simulink model "controlGPI_pos_6dof_conMI"  (R2023b)
settings: Solver=ode45  StartTime=0.0  StopTime=tsim  FixedStep=1e-4  MaxStep=tstep
undefined symbols (not defined in the file): contr_robot_params, ddq, dq, MI_Contr1, MI_Contr2, MI_Contr3, MI_Contr4, MI_Contr5, MI_Contr6, MI_motor1, MI_motor2, MI_motor3, MI_motor4, MI_motor5, MI_motor6, ndof, NN_Bspline_params, NN_RBF_params, nn_select, ns, Pc, q0, q_cero, q_eq, robot_params, sigbuilder_block, t_qeq_init, t_tr_init, t_trtr, tau_L, tau_L_mags, tr_muestra, tr_ref, Wc, Zc
libraries: mcbcontrolslib x12, spsRMSLib x12, simulink x2
(part 2 of 4)

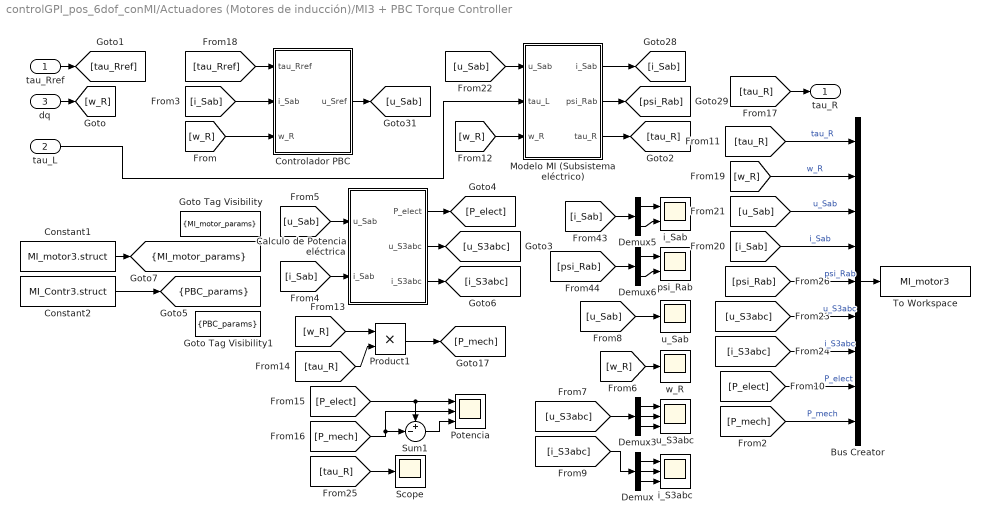
== system controlGPI_pos_6dof_conMI/Actuadores (Motores de inducción)/MI3 + PBC Torque Controller ==
  tau_Rref : Inport
  tau_L : Inport  Port=2
  dq : Inport  Port=3
  Bus Creator : BusCreator  Inputs=9
  Calculo de Potencia eléctrica : Subsystem
  Constant1 : Constant  Value=MI_motor3.struct  OutDataTypeStr=Bus: MI_bus
  Constant2 : Constant  Value=MI_Contr3.struct  OutDataTypeStr=Bus: Contr_bus
  Controlador PBC : Subsystem
  Demux : Demux  Outputs=3
  Demux3 : Demux  Outputs=3
  Demux5 : Demux  Outputs=2
  Demux6 : Demux  Outputs=2
  Goto Tag Visibility : GotoTagVisibility  GotoTag=MI_motor_params
  Goto Tag Visibility1 : GotoTagVisibility  GotoTag=PBC_params
  Modelo MI (Subsistema eléctrico) : Subsystem
  Potencia : Scope  NumInputPorts=3
  Product1 : Product
  Scope : Scope
  Sum1 : Sum  Inputs=+-|
  To Workspace : ToWorkspace  VariableName=MI_motor3  SaveFormat=Timeseries  SampleTime=-1
  i_S3abc : Scope  NumInputPorts=3
  i_Sab : Scope  NumInputPorts=2
  psi_Rab : Scope  NumInputPorts=2
  u_S3abc : Scope  NumInputPorts=3
  u_Sab : Scope
  w_R : Scope
  tau_R : Outport
  tag scope: MI_motor_params=scoped, PBC_params=scoped
  wires:
  Modelo MI (Subsistema eléctrico)/2(psi_Rab) -> [psi_Rab]
  [u_Sab] -> Modelo MI (Subsistema eléctrico)/1(u_Sab)
  [i_Sab] -> Controlador PBC/2(i_Sab)
  Controlador PBC/1(u_Sref) -> [u_Sab]
  [w_R] -> Controlador PBC/3(w_R)
  Calculo de Potencia eléctrica/2(u_S3abc) -> [u_S3abc]
  Calculo de Potencia eléctrica/1(P_elect) -> [P_elect]
  Demux5/1 -> i_Sab/1
  [w_R] -> w_R/1
  [u_Sab] -> Calculo de Potencia eléctrica/1(u_Sab)
  [psi_Rab] -> Demux6/1
  [u_Sab] -> u_Sab/1
  Demux6/1 -> psi_Rab/1
  Calculo de Potencia eléctrica/3(i_S3abc) -> [i_S3abc]
  Demux6/2 -> psi_Rab/2
  Demux5/2 -> i_Sab/2
  [i_Sab] -> Calculo de Potencia eléctrica/2(i_Sab)
  [i_Sab] -> Demux5/1
  Demux/2 -> i_S3abc/2
  Demux3/1 -> u_S3abc/1
  Demux3/3 -> u_S3abc/3
  [i_S3abc] -> Demux/1
  Demux/1 -> i_S3abc/1
  Demux/3 -> i_S3abc/3
  [u_S3abc] -> Demux3/1
  Demux3/2 -> u_S3abc/2
  Modelo MI (Subsistema eléctrico)/1(i_Sab) -> [i_Sab]
  Modelo MI (Subsistema eléctrico)/3(tau_R) -> [tau_R]
  Product1/1 -> [P_mech]
  [w_R] -> Product1/1
  [tau_R] -> Product1/2
  [tau_R] -> Bus Creator/1  "tau_R"
  Sum1/1 -> Potencia/3
  [P_elect] -> Potencia/1, Sum1/1
  [P_mech] -> Potencia/2, Sum1/2
  [tau_R] -> tau_R/1
  dq/1 -> [w_R]
  [tau_Rref] -> Controlador PBC/1(tau_Rref)
  [w_R] -> Modelo MI (Subsistema eléctrico)/3(w_R)
  Bus Creator/1 -> To Workspace/1
  Constant1/1 -> [MI_motor_params]
  [tau_R] -> Scope/1
  Constant2/1 -> [PBC_params]
  [w_R] -> Bus Creator/2  "w_R"
  [u_Sab] -> Bus Creator/3  "u_Sab"
  [i_Sab] -> Bus Creator/4  "i_Sab"
  [u_S3abc] -> Bus Creator/6  "u_S3abc"
  [i_S3abc] -> Bus Creator/7  "i_S3abc"
  [P_elect] -> Bus Creator/8  "P_elect"
  [P_mech] -> Bus Creator/9  "P_mech"
  tau_Rref/1 -> [tau_Rref]
  [psi_Rab] -> Bus Creator/5  "psi_Rab"
  tau_L/1 -> Modelo MI (Subsistema eléctrico)/2(tau_L)

== system controlGPI_pos_6dof_conMI/Actuadores (Motores de inducción)/MI4 + PBC Torque Controller ==
  tau_Rref : Inport
  tau_L : Inport  Port=2
  dq : Inport  Port=3
  Bus Creator : BusCreator  Inputs=9
  Calculo de Potencia eléctrica : Subsystem
  Constant1 : Constant  Value=MI_motor4.struct  OutDataTypeStr=Bus: MI_bus
  Constant2 : Constant  Value=MI_Contr4.struct  OutDataTypeStr=Bus: Contr_bus
  Controlador PBC : Subsystem
  Demux : Demux  Outputs=3
  Demux3 : Demux  Outputs=3
  Demux5 : Demux  Outputs=2
  Demux6 : Demux  Outputs=2
  Goto Tag Visibility : GotoTagVisibility  GotoTag=MI_motor_params
  Goto Tag Visibility1 : GotoTagVisibility  GotoTag=PBC_params
  Modelo MI (Subsistema eléctrico) : Subsystem
  Potencia : Scope  NumInputPorts=3
  Product1 : Product
  Scope : Scope
  Sum1 : Sum  Inputs=+-|
  To Workspace : ToWorkspace  VariableName=MI_motor4  SaveFormat=Timeseries  SampleTime=-1
  i_S3abc : Scope  NumInputPorts=3
  i_Sab : Scope  NumInputPorts=2
  psi_Rab : Scope  NumInputPorts=2
  u_S3abc : Scope  NumInputPorts=3
  u_Sab : Scope
  w_R : Scope
  tau_R : Outport
  tag scope: MI_motor_params=scoped, PBC_params=scoped
  wires:
  Modelo MI (Subsistema eléctrico)/2(psi_Rab) -> [psi_Rab]
  [u_Sab] -> Modelo MI (Subsistema eléctrico)/1(u_Sab)
  [i_Sab] -> Controlador PBC/2(i_Sab)
  Controlador PBC/1(u_Sref) -> [u_Sab]
  [w_R] -> Controlador PBC/3(w_R)
  Calculo de Potencia eléctrica/2(u_S3abc) -> [u_S3abc]
  Calculo de Potencia eléctrica/1(P_elect) -> [P_elect]
  Demux5/1 -> i_Sab/1
  [w_R] -> w_R/1
  [u_Sab] -> Calculo de Potencia eléctrica/1(u_Sab)
  [psi_Rab] -> Demux6/1
  [u_Sab] -> u_Sab/1
  Demux6/1 -> psi_Rab/1
  Calculo de Potencia eléctrica/3(i_S3abc) -> [i_S3abc]
  Demux6/2 -> psi_Rab/2
  Demux5/2 -> i_Sab/2
  [i_Sab] -> Calculo de Potencia eléctrica/2(i_Sab)
  [i_Sab] -> Demux5/1
  Demux/2 -> i_S3abc/2
  Demux3/1 -> u_S3abc/1
  Demux3/3 -> u_S3abc/3
  [i_S3abc] -> Demux/1
  Demux/1 -> i_S3abc/1
  Demux/3 -> i_S3abc/3
  [u_S3abc] -> Demux3/1
  Demux3/2 -> u_S3abc/2
  Modelo MI (Subsistema eléctrico)/1(i_Sab) -> [i_Sab]
  Modelo MI (Subsistema eléctrico)/3(tau_R) -> [tau_R]
  Product1/1 -> [P_mech]
  [w_R] -> Product1/1
  [tau_R] -> Product1/2
  [tau_R] -> Bus Creator/1  "tau_R"
  Sum1/1 -> Potencia/3
  [P_elect] -> Potencia/1, Sum1/1
  [P_mech] -> Potencia/2, Sum1/2
  [tau_R] -> tau_R/1
  dq/1 -> [w_R]
  [tau_Rref] -> Controlador PBC/1(tau_Rref)
  [w_R] -> Modelo MI (Subsistema eléctrico)/3(w_R)
  Bus Creator/1 -> To Workspace/1
  Constant1/1 -> [MI_motor_params]
  [tau_R] -> Scope/1
  Constant2/1 -> [PBC_params]
  [w_R] -> Bus Creator/2  "w_R"
  [u_Sab] -> Bus Creator/3  "u_Sab"
  [i_Sab] -> Bus Creator/4  "i_Sab"
  [u_S3abc] -> Bus Creator/6  "u_S3abc"
  [i_S3abc] -> Bus Creator/7  "i_S3abc"
  [P_elect] -> Bus Creator/8  "P_elect"
  [P_mech] -> Bus Creator/9  "P_mech"
  tau_Rref/1 -> [tau_Rref]
  [psi_Rab] -> Bus Creator/5  "psi_Rab"
  tau_L/1 -> Modelo MI (Subsistema eléctrico)/2(tau_L)

== system controlGPI_pos_6dof_conMI/Actuadores (Motores de inducción)/MI5 + PBC Torque Controller ==
  tau_Rref : Inport
  tau_L : Inport  Port=2
  dq : Inport  Port=3
  Bus Creator : BusCreator  Inputs=9
  Calculo de Potencia eléctrica : Subsystem
  Constant1 : Constant  Value=MI_motor5.struct  OutDataTypeStr=Bus: MI_bus
  Constant2 : Constant  Value=MI_Contr5.struct  OutDataTypeStr=Bus: Contr_bus
  Controlador PBC : Subsystem
  Demux : Demux  Outputs=3
  Demux3 : Demux  Outputs=3
  Demux5 : Demux  Outputs=2
  Demux6 : Demux  Outputs=2
  Goto Tag Visibility : GotoTagVisibility  GotoTag=MI_motor_params
  Goto Tag Visibility1 : GotoTagVisibility  GotoTag=PBC_params
  Modelo MI (Subsistema eléctrico) : Subsystem
  Potencia : Scope  NumInputPorts=3
  Product1 : Product
  Scope : Scope
  Sum1 : Sum  Inputs=+-|
  To Workspace : ToWorkspace  VariableName=MI_motor5  SaveFormat=Timeseries  SampleTime=-1
  i_S3abc : Scope  NumInputPorts=3
  i_Sab : Scope  NumInputPorts=2
  psi_Rab : Scope  NumInputPorts=2
  u_S3abc : Scope  NumInputPorts=3
  u_Sab : Scope
  w_R : Scope
  tau_R : Outport
  tag scope: MI_motor_params=scoped, PBC_params=scoped
  wires:
  Modelo MI (Subsistema eléctrico)/2(psi_Rab) -> [psi_Rab]
  [u_Sab] -> Modelo MI (Subsistema eléctrico)/1(u_Sab)
  [i_Sab] -> Controlador PBC/2(i_Sab)
  Controlador PBC/1(u_Sref) -> [u_Sab]
  [w_R] -> Controlador PBC/3(w_R)
  Calculo de Potencia eléctrica/2(u_S3abc) -> [u_S3abc]
  Calculo de Potencia eléctrica/1(P_elect) -> [P_elect]
  Demux5/1 -> i_Sab/1
  [w_R] -> w_R/1
  [u_Sab] -> Calculo de Potencia eléctrica/1(u_Sab)
  [psi_Rab] -> Demux6/1
  [u_Sab] -> u_Sab/1
  Demux6/1 -> psi_Rab/1
  Calculo de Potencia eléctrica/3(i_S3abc) -> [i_S3abc]
  Demux6/2 -> psi_Rab/2
  Demux5/2 -> i_Sab/2
  [i_Sab] -> Calculo de Potencia eléctrica/2(i_Sab)
  [i_Sab] -> Demux5/1
  Demux/2 -> i_S3abc/2
  Demux3/1 -> u_S3abc/1
  Demux3/3 -> u_S3abc/3
  [i_S3abc] -> Demux/1
  Demux/1 -> i_S3abc/1
  Demux/3 -> i_S3abc/3
  [u_S3abc] -> Demux3/1
  Demux3/2 -> u_S3abc/2
  Modelo MI (Subsistema eléctrico)/1(i_Sab) -> [i_Sab]
  Modelo MI (Subsistema eléctrico)/3(tau_R) -> [tau_R]
  Product1/1 -> [P_mech]
  [w_R] -> Product1/1
  [tau_R] -> Product1/2
  [tau_R] -> Bus Creator/1  "tau_R"
  Sum1/1 -> Potencia/3
  [P_elect] -> Potencia/1, Sum1/1
  [P_mech] -> Potencia/2, Sum1/2
  [tau_R] -> tau_R/1
  dq/1 -> [w_R]
  [tau_Rref] -> Controlador PBC/1(tau_Rref)
  [w_R] -> Modelo MI (Subsistema eléctrico)/3(w_R)
  Bus Creator/1 -> To Workspace/1
  Constant1/1 -> [MI_motor_params]
  [tau_R] -> Scope/1
  Constant2/1 -> [PBC_params]
  [w_R] -> Bus Creator/2  "w_R"
  [u_Sab] -> Bus Creator/3  "u_Sab"
  [i_Sab] -> Bus Creator/4  "i_Sab"
  [u_S3abc] -> Bus Creator/6  "u_S3abc"
  [i_S3abc] -> Bus Creator/7  "i_S3abc"
  [P_elect] -> Bus Creator/8  "P_elect"
  [P_mech] -> Bus Creator/9  "P_mech"
  tau_Rref/1 -> [tau_Rref]
  [psi_Rab] -> Bus Creator/5  "psi_Rab"
  tau_L/1 -> Modelo MI (Subsistema eléctrico)/2(tau_L)

== system controlGPI_pos_6dof_conMI/Actuadores (Motores de inducción)/MI6 + PBC Torque Controller ==
  tau_Rref : Inport
  tau_L : Inport  Port=2
  dq : Inport  Port=3
  Bus Creator : BusCreator  Inputs=9
  Calculo de Potencia eléctrica : Subsystem
  Constant1 : Constant  Value=MI_motor6.struct  OutDataTypeStr=Bus: MI_bus
  Constant2 : Constant  Value=MI_Contr6.struct  OutDataTypeStr=Bus: Contr_bus
  Controlador PBC : Subsystem
  Demux : Demux  Outputs=3
  Demux3 : Demux  Outputs=3
  Demux5 : Demux  Outputs=2
  Demux6 : Demux  Outputs=2
  Goto Tag Visibility : GotoTagVisibility  GotoTag=MI_motor_params
  Goto Tag Visibility1 : GotoTagVisibility  GotoTag=PBC_params
  Modelo MI (Subsistema eléctrico) : Subsystem
  Potencia : Scope  NumInputPorts=3
  Product1 : Product
  Scope : Scope
  Sum1 : Sum  Inputs=+-|
  To Workspace : ToWorkspace  VariableName=MI_motor6  SaveFormat=Timeseries  SampleTime=-1
  i_S3abc : Scope  NumInputPorts=3
  i_Sab : Scope  NumInputPorts=2
  psi_Rab : Scope  NumInputPorts=2
  u_S3abc : Scope  NumInputPorts=3
  u_Sab : Scope
  w_R : Scope
  tau_R : Outport
  tag scope: MI_motor_params=scoped, PBC_params=scoped
  wires:
  Modelo MI (Subsistema eléctrico)/2(psi_Rab) -> [psi_Rab]
  [u_Sab] -> Modelo MI (Subsistema eléctrico)/1(u_Sab)
  [i_Sab] -> Controlador PBC/2(i_Sab)
  Controlador PBC/1(u_Sref) -> [u_Sab]
  [w_R] -> Controlador PBC/3(w_R)
  Calculo de Potencia eléctrica/2(u_S3abc) -> [u_S3abc]
  Calculo de Potencia eléctrica/1(P_elect) -> [P_elect]
  Demux5/1 -> i_Sab/1
  [w_R] -> w_R/1
  [u_Sab] -> Calculo de Potencia eléctrica/1(u_Sab)
  [psi_Rab] -> Demux6/1
  [u_Sab] -> u_Sab/1
  Demux6/1 -> psi_Rab/1
  Calculo de Potencia eléctrica/3(i_S3abc) -> [i_S3abc]
  Demux6/2 -> psi_Rab/2
  Demux5/2 -> i_Sab/2
  [i_Sab] -> Calculo de Potencia eléctrica/2(i_Sab)
  [i_Sab] -> Demux5/1
  Demux/2 -> i_S3abc/2
  Demux3/1 -> u_S3abc/1
  Demux3/3 -> u_S3abc/3
  [i_S3abc] -> Demux/1
  Demux/1 -> i_S3abc/1
  Demux/3 -> i_S3abc/3
  [u_S3abc] -> Demux3/1
  Demux3/2 -> u_S3abc/2
  Modelo MI (Subsistema eléctrico)/1(i_Sab) -> [i_Sab]
  Modelo MI (Subsistema eléctrico)/3(tau_R) -> [tau_R]
  Product1/1 -> [P_mech]
  [w_R] -> Product1/1
  [tau_R] -> Product1/2
  [tau_R] -> Bus Creator/1  "tau_R"
  Sum1/1 -> Potencia/3
  [P_elect] -> Potencia/1, Sum1/1
  [P_mech] -> Potencia/2, Sum1/2
  [tau_R] -> tau_R/1
  dq/1 -> [w_R]
  [tau_Rref] -> Controlador PBC/1(tau_Rref)
  [w_R] -> Modelo MI (Subsistema eléctrico)/3(w_R)
  Bus Creator/1 -> To Workspace/1
  Constant1/1 -> [MI_motor_params]
  [tau_R] -> Scope/1
  Constant2/1 -> [PBC_params]
  [w_R] -> Bus Creator/2  "w_R"
  [u_Sab] -> Bus Creator/3  "u_Sab"
  [i_Sab] -> Bus Creator/4  "i_Sab"
  [u_S3abc] -> Bus Creator/6  "u_S3abc"
  [i_S3abc] -> Bus Creator/7  "i_S3abc"
  [P_elect] -> Bus Creator/8  "P_elect"
  [P_mech] -> Bus Creator/9  "P_mech"
  tau_Rref/1 -> [tau_Rref]
  [psi_Rab] -> Bus Creator/5  "psi_Rab"
  tau_L/1 -> Modelo MI (Subsistema eléctrico)/2(tau_L)

== system controlGPI_pos_6dof_conMI/ControladorGPI + NN/2 to 3 (1) ==
  In1 : Inport
  In2 : Inport  Port=2
  Demux : Demux  Outputs=3
  Demux1 : Demux  Outputs=3
  Mux : Mux  Inputs=2
  Mux1 : Mux  Inputs=2
  Mux2 : Mux  Inputs=2
  Out1 : Outport
  Out2 : Outport  Port=2
  Out3 : Outport  Port=3
  wires:
  Demux/3 -> Mux2/1
  Mux2/1 -> Out3/1
  Mux1/1 -> Out2/1
  Demux/1 -> Mux/1
  Demux1/1 -> Mux/2
  In1/1 -> Demux/1
  Demux/2 -> Mux1/1
  Demux1/2 -> Mux1/2
  Mux/1 -> Out1/1
  Demux1/3 -> Mux2/2
  In2/1 -> Demux1/1

== system controlGPI_pos_6dof_conMI/ControladorGPI + NN/3 to 6 (1)1 ==
  In1 : Inport
  In2 : Inport  Port=2
  In3 : Inport  Port=3
  Demux4 : Demux  Outputs=6
  Demux6 : Demux  Outputs=6
  Demux7 : Demux  Outputs=6
  Mux{,1..5} (6 alike) : Mux  Inputs=3
  Out1 : Outport
  Out2 : Outport  Port=2
  Out3 : Outport  Port=3
  Out4 : Outport  Port=4
  Out5 : Outport  Port=5
  Out6 : Outport  Port=6
  wires:
  Demux6/1 -> Mux2/1
  Demux6/3 -> Mux2/3
  Demux4/2 -> Mux/2
  Demux6/6 -> Mux3/3
  Demux6/2 -> Mux2/2
  Demux6/5 -> Mux3/2
  Mux/1 -> Out1/1
  In1/1 -> Demux4/1
  Demux6/4 -> Mux3/1
  Demux4/1 -> Mux/1
  Demux4/6 -> Mux1/3
  Demux4/4 -> Mux1/1
  Demux7/5 -> Mux5/2
  Demux4/3 -> Mux/3
  Demux4/5 -> Mux1/2
  Demux7/3 -> Mux4/3
  Demux7/1 -> Mux4/1
  Demux7/2 -> Mux4/2
  In3/1 -> Demux7/1
  Mux2/1 -> Out2/1
  Demux7/4 -> Mux5/1
  Demux7/6 -> Mux5/3
  In2/1 -> Demux6/1
  Mux5/1 -> Out6/1
  Mux1/1 -> Out4/1
  Mux4/1 -> Out3/1
  Mux3/1 -> Out5/1

== system controlGPI_pos_6dof_conMI/ControladorGPI + NN/3 to 9 (6) ==
  In1 : Inport
  In2 : Inport  Port=2
  In3 : Inport  Port=3
  Demux2 : Demux  Outputs=3
  Demux3 : Demux  Outputs=3
  Demux4 : Demux  Outputs=3
  Out1 : Outport
  Out2 : Outport  Port=2
  Out3 : Outport  Port=3
  Out4 : Outport  Port=4
  Out5 : Outport  Port=5
  Out6 : Outport  Port=6
  Out7 : Outport  Port=7
  Out8 : Outport  Port=8
  Out9 : Outport  Port=9
  wires:
  In3/1 -> Demux4/1
  Demux4/1 -> Out3/1
  Demux2/1 -> Out1/1
  Demux3/3 -> Out8/1
  Demux3/2 -> Out5/1
  Demux3/1 -> Out2/1
  In1/1 -> Demux2/1
  Demux2/3 -> Out7/1
  Demux4/3 -> Out9/1
  Demux4/2 -> Out6/1
  Demux2/2 -> Out4/1
  In2/1 -> Demux3/1

== system controlGPI_pos_6dof_conMI/ControladorGPI + NN/3 to 9 (7) ==
  In1 : Inport
  In2 : Inport  Port=2
  In3 : Inport  Port=3
  Demux2 : Demux  Outputs=3
  Demux3 : Demux  Outputs=3
  Demux4 : Demux  Outputs=3
  Out1 : Outport
  Out2 : Outport  Port=2
  Out3 : Outport  Port=3
  Out4 : Outport  Port=4
  Out5 : Outport  Port=5
  Out6 : Outport  Port=6
  Out7 : Outport  Port=7
  Out8 : Outport  Port=8
  Out9 : Outport  Port=9
  wires:
  In3/1 -> Demux4/1
  Demux4/1 -> Out3/1
  Demux2/1 -> Out1/1
  Demux3/3 -> Out8/1
  Demux3/2 -> Out5/1
  Demux3/1 -> Out2/1
  In1/1 -> Demux2/1
  Demux2/3 -> Out7/1
  Demux4/3 -> Out9/1
  Demux4/2 -> Out6/1
  Demux2/2 -> Out4/1
  In2/1 -> Demux3/1

== system controlGPI_pos_6dof_conMI/ControladorGPI + NN/Red neuronal ==
  q : Inport
  de_q : Inport  Port=2
  e_p : Inport  Port=3
  B-Spline NNs : Subsystem  TreatAsAtomicUnit=on
  Constant3 : Constant  Value=nn_select
  Constants : Subsystem  TreatAsAtomicUnit=on
  GPI_params : Scope  NumInputPorts=3
  Merge : Merge  Inputs=3
  Merge1 : Merge  Inputs=3
  Merge2 : Merge  Inputs=3
  RBF NNs : Subsystem  TreatAsAtomicUnit=on
  nn_select : Display
  param sintonization selector : If  IfExpression=u1 == 1  ElseIfExpressions=u1 == 2
  Wc : Outport
  Zc : Outport  Port=2
  Pc : Outport  Port=3
  wires:
  param sintonization selector/1 -> B-Spline NNs/Action
  B-Spline NNs/1(Wc) -> Merge/1
  param sintonization selector/3 -> Constants/Action
  Constant3/1 -> nn_select/1, param sintonization selector/1
  B-Spline NNs/2(Zc) -> Merge1/1
  B-Spline NNs/3(Pc) -> Merge2/1
  Constants/1(Wc) -> Merge/2
  Constants/2(Zc) -> Merge1/2
  Constants/3(Pc) -> Merge2/2
  q/1 -> [e_q]
  de_q/1 -> [de_q]
  param sintonization selector/2 -> RBF NNs/Action
  RBF NNs/2(Zc) -> Merge1/3
  RBF NNs/1(Wc) -> Merge/3
  RBF NNs/3(Pc) -> Merge2/3
  Merge/1 -> GPI_params/1, Wc/1
  Merge1/1 -> GPI_params/2, Zc/1
  Merge2/1 -> GPI_params/3, Pc/1
  [e_q] -> B-Spline NNs/1(e_q)
  [de_q] -> B-Spline NNs/2(de_q)
  [e_q] -> RBF NNs/1(e_q)
  [de_q] -> RBF NNs/2(de_q)
  e_p/1 -> [e_p]
  [e_p] -> RBF NNs/3(e_p)
  [e_p] -> B-Spline NNs/3(e_p)

== system controlGPI_pos_6dof_conMI/Perfil torque de carga tau_L/If Action Subsystem ==
  perfil_params : Inport
  Action Port : ActionPort  ActionPortLabel=elseif(u1 == 4)
  Clock2 : Clock
  Clock4 : Clock
  Polinomio 7mo orden sen : MATLAB Function  TreatAsAtomicUnit=on
  Scope1 : Scope
  Scope4 : Scope
  Scope5 : Scope  NumInputPorts=4
  Senoidal tiempo de inicio : MATLAB Function  TreatAsAtomicUnit=on
  Sum1 : Sum  Inputs=|-+
  senoidal : Sin  TimeSource=Use external signal  Frequency=6.2832  Phase=1.5708  SampleTime=0
  sen : Outport
  wires:
  Clock4/1 -> Polinomio 7mo orden sen/1(t)
  Polinomio 7mo orden sen/1(qpol) -> Scope1/1, Sum1/1, Scope5/1
  Sum1/1 -> Scope4/1, [sen]
  Polinomio 7mo orden sen/4(jpol) -> Scope5/4
  Polinomio 7mo orden sen/3(apol) -> Scope5/3
  Clock2/1 -> Senoidal tiempo de inicio/1(t)
  [perfil_params] -> Polinomio 7mo orden sen/2(perfil_params)
  Polinomio 7mo orden sen/2(vpol) -> Scope5/2
  senoidal/1 -> Sum1/2
  Senoidal tiempo de inicio/1(tr) -> senoidal/1
  [sen] -> sen/1
  perfil_params/1 -> [perfil_params]
  [perfil_params] -> Senoidal tiempo de inicio/2(perfil_params)

== system controlGPI_pos_6dof_conMI/Perfil torque de carga tau_L/If Action Subsystem1 ==
  Action Port : ActionPort  ActionPortLabel=if(u1 == 1)
  Constant : Constant  Value=0
  cero : Outport
  wires:
  Constant/1 -> cero/1

== system controlGPI_pos_6dof_conMI/Perfil torque de carga tau_L/If Action Subsystem2 ==
  Action Port : ActionPort  ActionPortLabel=elseif(u1 == 2)
  Scope3 : Scope
  Sum : Sum  Inputs=|++
  escalon1 : Step  Time=2.5  After=0.70582  SampleTime=0
  escalon2 : Step  Time=7.5  After=-0.70582  SampleTime=0
  esca : Outport
  wires:
  escalon2/1 -> Sum/2
  escalon1/1 -> Sum/1
  Sum/1 -> [esca], Scope3/1
  [esca] -> esca/1

== system controlGPI_pos_6dof_conMI/Perfil torque de carga tau_L/If Action Subsystem3 ==
  Action Port : ActionPort  ActionPortLabel=elseif(u1 == 3)
  Scope2 : Scope
  Sum2 : Sum  Inputs=|++
  rampa1 : simulink/Sources/Ramp  slope=0.02064  start=2.5  InitialOutput=0
  rampa2 : simulink/Sources/Ramp  slope=-0.02064  start=7.5  InitialOutput=0
  ramp : Outport
  wires:
  rampa2/1 -> Sum2/2
  rampa1/1 -> Sum2/1
  Sum2/1 -> Scope2/1, [ramp]
  [ramp] -> ramp/1

== system controlGPI_pos_6dof_conMI/Perfil torque de carga tau_L/If Action Subsystem4 ==
  perfil_params : Inport
  Action Port : ActionPort  ActionPortLabel=elseif(u1 == 5)
  Clock1 : Clock
  Polinomio 7mo orden tau_L : MATLAB Function  TreatAsAtomicUnit=on
  Scope : Scope  NumInputPorts=4
  pol7 : Outport
  wires:
  Polinomio 7mo orden tau_L/4(jpol) -> Scope/4
  Polinomio 7mo orden tau_L/1(qpol) -> Scope/1, [pol7]
  Polinomio 7mo orden tau_L/2(vpol) -> Scope/2
  Clock1/1 -> Polinomio 7mo orden tau_L/1(t)
  Polinomio 7mo orden tau_L/3(apol) -> Scope/3
  perfil_params/1 -> Polinomio 7mo orden tau_L/2(perfil_params)
  [pol7] -> pol7/1

== system controlGPI_pos_6dof_conMI/Perfil torque de carga tau_L/If Action Subsystem5 ==
  perfil_params : Inport
  Action Port : ActionPort  ActionPortLabel=elseif(u1 == 6)
  Clock : Clock
  Scope1 : Scope
  Tren de esca : MATLAB Function  TreatAsAtomicUnit=on
  trEsca : Outport
  wires:
  Tren de esca/1(q) -> Scope1/1, [trEsca]
  Clock/1 -> Tren de esca/1(t)
  perfil_params/1 -> Tren de esca/2(perfil_params)
  [trEsca] -> trEsca/1

== system controlGPI_pos_6dof_conMI/Perfil torque de carga tau_L/If Action Subsystem6 ==
  Action Port : ActionPort  ActionPortLabel=elseif(u1 == 7)
  Clock3 : Clock
  Polinomio 7mo orden timeseries : MATLAB Function  TreatAsAtomicUnit=on
  Product : Product
  Scope6 : Scope  NumInputPorts=4
  ts_data1 : FromWorkspace  Commented=on  VariableName=tau_L_ts
  ts : Outport
  wires:
  Product/1 -> [ts]
  Clock3/1 -> Polinomio 7mo orden timeseries/1(t)
  ts_data1/1 -> Product/1
  Polinomio 7mo orden timeseries/4(jpol) -> Scope6/4
  Polinomio 7mo orden timeseries/2(vpol) -> Scope6/2
  Polinomio 7mo orden timeseries/3(apol) -> Scope6/3
  Polinomio 7mo orden timeseries/1(qpol) -> Product/2, Scope6/1
  [ts] -> ts/1

== system controlGPI_pos_6dof_conMI/Perfil torque de carga tau_L/If Action Subsystem7 ==
  perfil_params : Inport
  Action Port : ActionPort  ActionPortLabel=elseif(u1 == 8)
  Clock5 : Clock
  Scope7 : Scope
  Trayectoria 15 segmentos : MATLAB Function  TreatAsAtomicUnit=on
  tr15segs : Outport
  wires:
  Clock5/1 -> Trayectoria 15 segmentos/1(t)
  Trayectoria 15 segmentos/1(q) -> Scope7/1, [tr15segs]
  [tr15segs] -> tr15segs/1
  perfil_params/1 -> Trayectoria 15 segmentos/2(perfil_params)

== system controlGPI_pos_6dof_conMI/Trayectoria de referencia/2 to 3 (2) ==
  In1 : Inport
  In2 : Inport  Port=2
  Demux3 : Demux  Outputs=3
  Demux4 : Demux  Outputs=3
  Mux10 : Mux  Inputs=2
  Mux8 : Mux  Inputs=2
  Mux9 : Mux  Inputs=2
  1 : Outport
  2 : Outport  Port=2
  3 : Outport  Port=3
  wires:
  Demux4/3 -> Mux10/2
  Demux3/1 -> Mux8/1
  Demux3/2 -> Mux9/1
  Mux9/1 -> 2/1
  Demux4/2 -> Mux9/2
  Demux4/1 -> Mux8/2
  Demux3/3 -> Mux10/1
  Mux8/1 -> 1/1
  Mux10/1 -> 3/1
  In1/1 -> Demux3/1
  In2/1 -> Demux4/1

== system controlGPI_pos_6dof_conMI/Trayectoria de referencia/2 to 3 (2)1 ==
  In1 : Inport
  In2 : Inport  Port=2
  Demux3 : Demux  Outputs=3
  Demux4 : Demux  Outputs=3
  Mux10 : Mux  Inputs=2
  Mux8 : Mux  Inputs=2
  Mux9 : Mux  Inputs=2
  1 : Outport
  2 : Outport  Port=2
  3 : Outport  Port=3
  wires:
  Demux4/3 -> Mux10/2
  Demux3/1 -> Mux8/1
  Demux3/2 -> Mux9/1
  Mux9/1 -> 2/1
  Demux4/2 -> Mux9/2
  Demux4/1 -> Mux8/2
  Demux3/3 -> Mux10/1
  Mux8/1 -> 1/1
  Mux10/1 -> 3/1
  In1/1 -> Demux3/1
  In2/1 -> Demux4/1

== system controlGPI_pos_6dof_conMI/Trayectoria de referencia/2 to 3 (2)2 ==
  In1 : Inport
  In2 : Inport  Port=2
  Demux3 : Demux  Outputs=3
  Demux4 : Demux  Outputs=3
  Mux10 : Mux  Inputs=2
  Mux8 : Mux  Inputs=2
  Mux9 : Mux  Inputs=2
  1 : Outport
  2 : Outport  Port=2
  3 : Outport  Port=3
  wires:
  Demux4/3 -> Mux10/2
  Demux3/1 -> Mux8/1
  Demux3/2 -> Mux9/1
  Mux9/1 -> 2/1
  Demux4/2 -> Mux9/2
  Demux4/1 -> Mux8/2
  Demux3/3 -> Mux10/1
  Mux8/1 -> 1/1
  Mux10/1 -> 3/1
  In1/1 -> Demux3/1
  In2/1 -> Demux4/1

== system controlGPI_pos_6dof_conMI/Trayectoria de referencia/3 to 6 (1) ==
  In1 : Inport
  In2 : Inport  Port=2
  In3 : Inport  Port=3
  Demux4 : Demux  Outputs=6
  Demux6 : Demux  Outputs=6
  Demux7 : Demux  Outputs=6
  Mux{,1..5} (6 alike) : Mux  Inputs=3
  Out1 : Outport
  Out2 : Outport  Port=2
  Out3 : Outport  Port=3
  Out4 : Outport  Port=4
  Out5 : Outport  Port=5
  Out6 : Outport  Port=6
  wires:
  Demux6/1 -> Mux2/1
  Demux6/3 -> Mux2/3
  Demux4/2 -> Mux/2
  Demux6/6 -> Mux3/3
  Demux6/2 -> Mux2/2
  Demux6/5 -> Mux3/2
  Mux/1 -> Out1/1
  In1/1 -> Demux4/1
  Demux6/4 -> Mux3/1
  Demux4/1 -> Mux/1
  Demux4/6 -> Mux1/3
  Demux4/4 -> Mux1/1
  Demux7/5 -> Mux5/2
  Demux4/3 -> Mux/3
  Demux4/5 -> Mux1/2
  Demux7/3 -> Mux4/3
  Demux7/1 -> Mux4/1
  Demux7/2 -> Mux4/2
  In3/1 -> Demux7/1
  Mux2/1 -> Out2/1
  Demux7/4 -> Mux5/1
  Demux7/6 -> Mux5/3
  In2/1 -> Demux6/1
  Mux5/1 -> Out6/1
  Mux1/1 -> Out4/1
  Mux4/1 -> Out3/1
  Mux3/1 -> Out5/1

== system controlGPI_pos_6dof_conMI/Trayectoria de referencia/3 to 9 (4) ==
  In1 : Inport
  In2 : Inport  Port=2
  In3 : Inport  Port=3
  Demux2 : Demux  Outputs=3
  Demux3 : Demux  Outputs=3
  Demux4 : Demux  Outputs=3
  Out1 : Outport
  Out2 : Outport  Port=2
  Out3 : Outport  Port=3
  Out4 : Outport  Port=4
  Out5 : Outport  Port=5
  Out6 : Outport  Port=6
  Out7 : Outport  Port=7
  Out8 : Outport  Port=8
  Out9 : Outport  Port=9
  wires:
  In3/1 -> Demux4/1
  Demux4/1 -> Out3/1
  Demux2/1 -> Out1/1
  Demux3/3 -> Out8/1
  Demux3/2 -> Out5/1
  Demux3/1 -> Out2/1
  In1/1 -> Demux2/1
  Demux2/3 -> Out7/1
  Demux4/3 -> Out9/1
  Demux4/2 -> Out6/1
  Demux2/2 -> Out4/1
  In2/1 -> Demux3/1

== system controlGPI_pos_6dof_conMI/Trayectoria de referencia/3 to 9 (5) ==
  In1 : Inport
  In2 : Inport  Port=2
  In3 : Inport  Port=3
  Demux2 : Demux  Outputs=3
  Demux3 : Demux  Outputs=3
  Demux4 : Demux  Outputs=3
  Out1 : Outport
  Out2 : Outport  Port=2
  Out3 : Outport  Port=3
  Out4 : Outport  Port=4
  Out5 : Outport  Port=5
  Out6 : Outport  Port=6
  Out7 : Outport  Port=7
  Out8 : Outport  Port=8
  Out9 : Outport  Port=9
  wires:
  In3/1 -> Demux4/1
  Demux4/1 -> Out3/1
  Demux2/1 -> Out1/1
  Demux3/3 -> Out8/1
  Demux3/2 -> Out5/1
  Demux3/1 -> Out2/1
  In1/1 -> Demux2/1
  Demux2/3 -> Out7/1
  Demux4/3 -> Out9/1
  Demux4/2 -> Out6/1
  Demux2/2 -> Out4/1
  In2/1 -> Demux3/1

== system controlGPI_pos_6dof_conMI/Trayectoria de referencia/3 to 9 (7) ==
  In1 : Inport
  In2 : Inport  Port=2
  In3 : Inport  Port=3
  Demux2 : Demux  Outputs=3
  Demux3 : Demux  Outputs=3
  Demux4 : Demux  Outputs=3
  Out1 : Outport
  Out2 : Outport  Port=2
  Out3 : Outport  Port=3
  Out4 : Outport  Port=4
  Out5 : Outport  Port=5
  Out6 : Outport  Port=6
  Out7 : Outport  Port=7
  Out8 : Outport  Port=8
  Out9 : Outport  Port=9
  wires:
  In3/1 -> Demux4/1
  Demux4/1 -> Out3/1
  Demux2/1 -> Out1/1
  Demux3/3 -> Out8/1
  Demux3/2 -> Out5/1
  Demux3/1 -> Out2/1
  In1/1 -> Demux2/1
  Demux2/3 -> Out7/1
  Demux4/3 -> Out9/1
  Demux4/2 -> Out6/1
  Demux2/2 -> Out4/1
  In2/1 -> Demux3/1

== system controlGPI_pos_6dof_conMI/Trayectoria de referencia/Inicializar posición de robot manipulador ==
  q_r : Inport
  2 to 6 (3) : Subsystem
  Clock1 : Clock
  Constant : Constant  Value=q0
  Constant1 : Constant  Value=q_eq
  Constant2 : Constant  Value=tr_muestra
  Constant3 : Constant  Value=ndof
  Constant4 : Constant  Value=t_qeq_init
  Constant5 : Constant  Value=t_trtr
  Constant7 : Constant  Value=t_tr_init
  Demux{4..7} (4 alike) : Demux  Outputs=6
  Derivative : Derivative
  Derivative1 : Derivative
  ddq_ref1 : Scope  NumInputPorts=6
  dq_ref1 : Scope  NumInputPorts=6
  interp_pol7_q_r : MATLAB Function  TreatAsAtomicUnit=on
  q_r1 : Scope  NumInputPorts=6
  q_r_comp : Scope  NumInputPorts=6
  q_ref1 : Scope  NumInputPorts=6
  q_ref : Outport
  dq_ref : Outport  Port=2
  ddq_ref : Outport  Port=3
  wires:
  [ddq_ref] -> ddq_ref/1
  q_r/1 -> [q_r]
  [dq_ref] -> dq_ref/1
  [q_ref] -> q_ref/1
  2 to 6 (3)/1(Out1) -> q_r_comp/1
  [q_r] -> 2 to 6 (3)/1(In1)
  2 to 6 (3)/3(Out3) -> q_r_comp/3
  2 to 6 (3)/5(Out5) -> q_r_comp/5
  2 to 6 (3)/6(Out6) -> q_r_comp/6
  [q_ref] -> 2 to 6 (3)/2(In2)
  2 to 6 (3)/2(Out2) -> q_r_comp/2
  2 to 6 (3)/4(Out4) -> q_r_comp/4
  Demux4/3 -> q_r1/3
  Demux4/5 -> q_r1/5
  Demux4/4 -> q_r1/4
  Demux4/2 -> q_r1/2
  Demux4/6 -> q_r1/6
  Demux4/1 -> q_r1/1
  [q_r] -> Demux4/1
  Constant7/1 -> interp_pol7_q_r/6(t1)
  Clock1/1 -> interp_pol7_q_r/1(t)
  interp_pol7_q_r/1(interp_qpos) -> Derivative/1, [q_ref]
  Constant1/1 -> interp_pol7_q_r/2(q_eq)
  Constant/1 -> interp_pol7_q_r/3(q_cero)
  Derivative/1 -> [dq_ref], Derivative1/1
  Derivative1/1 -> [ddq_ref]
  Demux5/6 -> q_ref1/6
  Demux5/2 -> q_ref1/2
  [q_ref] -> Demux5/1
  Demux5/1 -> q_ref1/1
  Demux5/4 -> q_ref1/4
  Demux5/5 -> q_ref1/5
  Demux5/3 -> q_ref1/3
  Demux6/1 -> dq_ref1/1
  Demux6/4 -> dq_ref1/4
  Demux6/5 -> dq_ref1/5
  [dq_ref] -> Demux6/1
  Demux6/6 -> dq_ref1/6
  Demux6/2 -> dq_ref1/2
  Demux6/3 -> dq_ref1/3
  Demux7/2 -> ddq_ref1/2
  Demux7/4 -> ddq_ref1/4
  Demux7/3 -> ddq_ref1/3
  [ddq_ref] -> Demux7/1
  Demux7/1 -> ddq_ref1/1
  Demux7/6 -> ddq_ref1/6
  Demux7/5 -> ddq_ref1/5
  [q_r] -> interp_pol7_q_r/4(q_tr_init)
  Constant4/1 -> interp_pol7_q_r/5(t0)
  Constant2/1 -> interp_pol7_q_r/8(tr_muestra)
  Constant3/1 -> interp_pol7_q_r/9(ndof)
  Constant5/1 -> interp_pol7_q_r/7(t_trtr)

== system controlGPI_pos_6dof_conMI/Actuadores (Motores de inducción)/MI1 + PBC Torque Controller/Calculo de Potencia eléctrica ==
  u_Sab : Inport
  i_Sab : Inport  Port=2
  Demux1 : Demux  Commented=on  Outputs=3
  Demux2 : Demux  Commented=on  Outputs=3
  Demux3 : Demux  Commented=on  Outputs=3
  Demux4 : Demux  Outputs=3
  From1 : From  Commented=on  GotoTag=u_S3abc
  From2 : From  Commented=on  GotoTag=i_S3abc
  IIR Filter : mcbcontrolslib/IIR Filter  Commented=on  VariantControl=Low Pass Filter  VariantSelect=Low-pass  Filter_constant=0.04  advancedSettings=on  Ts=50e-6  cutOff_freq=132.6291
      settings: LibrarySourceBlock=mcbhdllib/Signal Management/IIR Filter
  IIR Filter1 : mcbcontrolslib/IIR Filter  Commented=on  VariantControl=Low Pass Filter  VariantSelect=Low-pass  Filter_constant=0.04  advancedSettings=on  Ts=50e-6  cutOff_freq=132.6291
      settings: LibrarySourceBlock=mcbhdllib/Signal Management/IIR Filter
  Product1 : Product
  Product2 : Product  Commented=on
  RMS : spsRMSLib/RMS  Commented=on  TrueRMS=on  Freq=60  RMSInit=120  Ts=0
  RMS1 : spsRMSLib/RMS  Commented=on  TrueRMS=on  Freq=60  RMSInit=120  Ts=0
  Scope : Scope  Commented=on
  Scope1 : Scope  Commented=on
  Scope11 : Scope  Commented=on
  Sum1 : Sum  Inputs=|+++
  Sum2 : Sum  Commented=on  Inputs=|+++
  ab0 - ABC : MATLAB Function  TreatAsAtomicUnit=on
  ab0 - ABC1 : MATLAB Function  TreatAsAtomicUnit=on
  i_S3abc1 : Scope  Commented=on  NumInputPorts=3
  u_S3abc1 : Scope  Commented=on  NumInputPorts=3
  P_elect : Outport
  u_S3abc : Outport  Port=2
  i_S3abc : Outport  Port=3
  wires:
  Sum1/1 -> P_elect/1
  Demux4/1 -> Sum1/1
  [i_S3abc] -> Product1/2
  i_Sab/1 -> ab0 - ABC1/1(BPu)
  Demux4/3 -> Sum1/3
  [u_S3abc] -> Product1/1
  Demux4/2 -> Sum1/2
  Product1/1 -> Demux4/1
  u_Sab/1 -> ab0 - ABC/1(BPu)
  [u_S3abc] -> u_S3abc/1
  [i_S3abc] -> i_S3abc/1
  ab0 - ABC/1(u) -> [u_S3abc]
  ab0 - ABC1/1(u) -> [i_S3abc]
  IIR Filter/1 -> Product2/1, Demux1/1
  RMS/1 -> Scope11/1
  Demux1/2 -> u_S3abc1/2
  Demux1/3 -> u_S3abc1/3
  Demux1/1 -> RMS/1, u_S3abc1/1
  From1/1 -> IIR Filter/1
  Demux2/1 -> RMS1/1, i_S3abc1/1
  RMS1/1 -> Scope1/1
  Demux2/2 -> i_S3abc1/2
  IIR Filter1/1 -> Product2/2, Demux2/1
  From2/1 -> IIR Filter1/1
  Demux2/3 -> i_S3abc1/3
  Demux3/2 -> Sum2/2
  Demux3/3 -> Sum2/3
  Sum2/1 -> Scope/1
  Product2/1 -> Demux3/1
  Demux3/1 -> Sum2/1

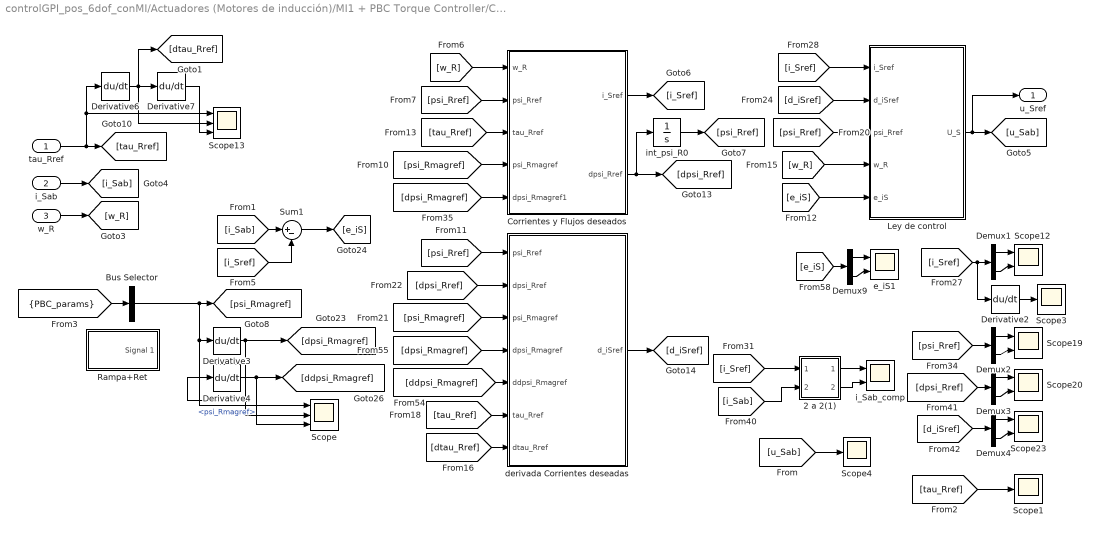
== system controlGPI_pos_6dof_conMI/Actuadores (Motores de inducción)/MI1 + PBC Torque Controller/Controlador PBC ==
  tau_Rref : Inport
  i_Sab : Inport  Port=2
  w_R : Inport  Port=3
  2 a 2(1) : Subsystem
  Bus Selector : BusSelector  OutputSignals=psi_Rmagref
  Corrientes y Flujos deseados : Subsystem
  Demux{1..4,9} (5 alike) : Demux  Outputs=2
  Derivative{2..4,6..7} (5 alike) : Derivative
  Ley de control : Subsystem
  Rampa+Ret : Subsystem  Tag=STV Subsys  LoadFcn=sigbuilder_block('load');  StartFcn=sigbuilder_block('start');  StopFcn=sigbuilder_block('stop');  ClipboardFcn=sigbuilder_block('clipboard');  mask(Sigbuilder block){tuvar=[0:10]}
      mask help: Sigbuilder GUI
      mask init:
      | if ~strcmp(get_param(bdroot(gcbh),'SimulationStatus'),'stopped') tuvar = sigbuilder_block('maskInit'); end
      settings: CopyFcn=sigbuilder_block('copy');  DeleteFcn=sigbuilder_block('delete');  ModelCloseFcn=sigbuilder_block('modelClose');  PreSaveFcn=sigbuilder_block('preSave');  PauseFcn=sigbuilder_block('pause')  ContinueFcn=sigbuilder_block('continue')  NameChangeFcn=sigbuilder_block('namechange');  OpenFcn=sigbuilder_block('open',[280.5 86.5 550.5 399.5 ]);  CloseFcn=sigbuilder_block('close');
      mask Display: plot(0, 0, 100, 100,[2, 2, 32, 32, 2], [68, 8, 8, 68, 68],[32, 2], [38, 38], [32, 19, 2],[53, 60, 44], [32, 17, 17, 2],[16, 16, 31, 31]);txt = getActiveGroup(gcbh);text(2, 100, txt,'verticalAlignment', 'top');
  Scope : Scope  NumInputPorts=3
  Scope1 : Scope
  Scope{12,19..20,23} (4 alike) : Scope  NumInputPorts=2
  Scope13 : Scope  NumInputPorts=3
  Scope3 : Scope
  Scope4 : Scope
  Sum1 : Sum  Inputs=|+-
  derivada Corrientes deseadas : Subsystem
  e_iS1 : Scope  NumInputPorts=2
  i_Sab_comp : Scope  NumInputPorts=2
  int_psi_R0 : Integrator  InitialCondition=[0.51032;0]
  u_Sref : Outport
  wires:
  Derivative3/1 -> Scope/2, Derivative4/1, [dpsi_Rmagref]
  Derivative4/1 -> [ddpsi_Rmagref], Scope/3
  Bus Selector/1 -> Scope/1, Derivative3/1, [psi_Rmagref]  "<psi_Rmagref>"
  i_Sab/1 -> [i_Sab]
  Demux1/1 -> Scope12/1
  [d_iSref] -> Demux4/1
  Demux3/2 -> Scope20/2
  Demux2/1 -> Scope19/1
  Demux1/2 -> Scope12/2
  [dpsi_Rref] -> Demux3/1
  Demux3/1 -> Scope20/1
  Demux4/1 -> Scope23/1
  [psi_Rref] -> Demux2/1
  Demux4/2 -> Scope23/2
  Demux2/2 -> Scope19/2
  [tau_Rref] -> Corrientes y Flujos deseados/3(tau_Rref)
  [w_R] -> Corrientes y Flujos deseados/1(w_R)
  int_psi_R0/1 -> [psi_Rref]
  Corrientes y Flujos deseados/2(dpsi_Rref) -> int_psi_R0/1, [dpsi_Rref]
  [psi_Rref] -> Corrientes y Flujos deseados/2(psi_Rref)
  [psi_Rmagref] -> Corrientes y Flujos deseados/4(psi_Rmagref)
  [dpsi_Rmagref] -> Corrientes y Flujos deseados/5(dpsi_Rmagref1)
  [psi_Rref] -> derivada Corrientes deseadas/1(psi_Rref)
  [dpsi_Rref] -> derivada Corrientes deseadas/2(dpsi_Rref)
  [psi_Rmagref] -> derivada Corrientes deseadas/3(psi_Rmagref)
  [dpsi_Rmagref] -> derivada Corrientes deseadas/4(dpsi_Rmagref)
  [ddpsi_Rmagref] -> derivada Corrientes deseadas/5(ddpsi_Rmagref)
  [tau_Rref] -> derivada Corrientes deseadas/6(tau_Rref)
  [dtau_Rref] -> derivada Corrientes deseadas/7(dtau_Rref)
  derivada Corrientes deseadas/1(d_iSref) -> [d_iSref]
  [e_iS] -> Demux9/1
  Demux9/1 -> e_iS1/1
  Demux9/2 -> e_iS1/2
  [i_Sab] -> Sum1/1
  [i_Sref] -> Sum1/2
  Sum1/1 -> [e_iS]
  [u_Sab] -> Scope4/1
  [i_Sref] -> Ley de control/1(i_Sref)
  [d_iSref] -> Ley de control/2(d_iSref)
  [psi_Rref] -> Ley de control/3(psi_Rref)
  [w_R] -> Ley de control/4(w_R)
  Ley de control/1(U_S) -> u_Sref/1, [u_Sab]
  [e_iS] -> Ley de control/5(e_iS)
  Derivative7/1 -> Scope13/3
  tau_Rref/1 -> Derivative6/1, Scope13/1, [tau_Rref]
  Derivative6/1 -> [dtau_Rref], Derivative7/1, Scope13/2
  2 a 2(1)/2(Out2) -> i_Sab_comp/2
  2 a 2(1)/1(Out1) -> i_Sab_comp/1
  [i_Sab] -> 2 a 2(1)/2(In2)
  [i_Sref] -> 2 a 2(1)/1(In1)
  [i_Sref] -> Derivative2/1, Demux1/1
  Derivative2/1 -> Scope3/1
  w_R/1 -> [w_R]
  [tau_Rref] -> Scope1/1
  [PBC_params] -> Bus Selector/1
  Corrientes y Flujos deseados/1(i_Sref) -> [i_Sref]

== system controlGPI_pos_6dof_conMI/Actuadores (Motores de inducción)/MI1 + PBC Torque Controller/Modelo MI (Subsistema eléctrico) ==
  u_Sab : Inport
  tau_L : Inport  Port=2
  w_R : Inport  Port=3
  Demux : Demux  Outputs=2
  Demux7 : Demux  Outputs=2
  Demux8 : Demux  Outputs=2
  Integrator : Integrator
  Integrator1 : Integrator
  Modelo Motor de inducción (Subsistema eléctrico) : MATLAB Function  TreatAsAtomicUnit=on
  Scope11 : Scope
  Scope3 : Scope  NumInputPorts=2
  Scope31 : Scope
  ab/dq : MATLAB Function  TreatAsAtomicUnit=on
  d_iSab : Scope  NumInputPorts=2
  dpsi_Rab1 : Scope  NumInputPorts=2
  i_Sab : Outport
  psi_Rab : Outport  Port=2
  tau_R : Outport  Port=3
  wires:
  Modelo Motor de inducción (Subsistema eléctrico)/1(di_Sab) -> Integrator/1, [d_iSab]
  Modelo Motor de inducción (Subsistema eléctrico)/2(dpsi_Rab) -> Integrator1/1, [dpsi_Rab]
  [w_R] -> Modelo Motor de inducción (Subsistema eléctrico)/5(w_R)
  [psi_Rab] -> Modelo Motor de inducción (Subsistema eléctrico)/4(psi_Rab)
  [i_Sab] -> Modelo Motor de inducción (Subsistema eléctrico)/3(i_Sab)
  Integrator1/1 -> [psi_Rab]
  u_Sab/1 -> [u_Sab]
  Modelo Motor de inducción (Subsistema eléctrico)/3(tau_R) -> [tau_R]
  [tau_R] -> Scope3/1
  ab/dq/1(psi_Rmag) -> Scope11/1
  [psi_Rab] -> Demux/1
  Demux7/1 -> dpsi_Rab1/1
  Demux7/2 -> dpsi_Rab1/2
  [d_iSab] -> Demux8/1
  ab/dq/2(rho) -> Scope31/1
  Demux/1 -> ab/dq/1(psi_ra)
  Demux8/2 -> d_iSab/2
  Demux8/1 -> d_iSab/1
  [dpsi_Rab] -> Demux7/1
  Demux/2 -> ab/dq/2(psi_rb)
  Integrator/1 -> [i_Sab]
  [MI_motor_params] -> Modelo Motor de inducción (Subsistema eléctrico)/1(MI_motor_params)
  [u_Sab] -> Modelo Motor de inducción (Subsistema eléctrico)/2(u_Sab)
  tau_L/1 -> [tau_L]
  [tau_L] -> Modelo Motor de inducción (Subsistema eléctrico)/6(tau_L)
  w_R/1 -> [w_R]
  [tau_R] -> tau_R/1
  [psi_Rab] -> psi_Rab/1
  [i_Sab] -> i_Sab/1
  [tau_L] -> Scope3/2

== system controlGPI_pos_6dof_conMI/Actuadores (Motores de inducción)/MI2 + PBC Torque Controller/Calculo de Potencia eléctrica ==
  u_Sab : Inport
  i_Sab : Inport  Port=2
  Demux1 : Demux  Commented=on  Outputs=3
  Demux2 : Demux  Commented=on  Outputs=3
  Demux3 : Demux  Commented=on  Outputs=3
  Demux4 : Demux  Outputs=3
  From1 : From  Commented=on  GotoTag=u_S3abc
  From2 : From  Commented=on  GotoTag=i_S3abc
  IIR Filter : mcbcontrolslib/IIR Filter  Commented=on  VariantControl=Low Pass Filter  VariantSelect=Low-pass  Filter_constant=0.04  advancedSettings=on  Ts=50e-6  cutOff_freq=132.6291
      settings: LibrarySourceBlock=mcbhdllib/Signal Management/IIR Filter
  IIR Filter1 : mcbcontrolslib/IIR Filter  Commented=on  VariantControl=Low Pass Filter  VariantSelect=Low-pass  Filter_constant=0.04  advancedSettings=on  Ts=50e-6  cutOff_freq=132.6291
      settings: LibrarySourceBlock=mcbhdllib/Signal Management/IIR Filter
  Product1 : Product
  Product2 : Product  Commented=on
  RMS : spsRMSLib/RMS  Commented=on  TrueRMS=on  Freq=60  RMSInit=120  Ts=0
  RMS1 : spsRMSLib/RMS  Commented=on  TrueRMS=on  Freq=60  RMSInit=120  Ts=0
  Scope : Scope  Commented=on
  Scope1 : Scope  Commented=on
  Scope11 : Scope  Commented=on
  Sum1 : Sum  Inputs=|+++
  Sum2 : Sum  Commented=on  Inputs=|+++
  ab0 - ABC : MATLAB Function  TreatAsAtomicUnit=on
  ab0 - ABC1 : MATLAB Function  TreatAsAtomicUnit=on
  i_S3abc1 : Scope  Commented=on  NumInputPorts=3
  u_S3abc1 : Scope  Commented=on  NumInputPorts=3
  P_elect : Outport
  u_S3abc : Outport  Port=2
  i_S3abc : Outport  Port=3
  wires:
  Sum1/1 -> P_elect/1
  Demux4/1 -> Sum1/1
  [i_S3abc] -> Product1/2
  i_Sab/1 -> ab0 - ABC1/1(BPu)
  Demux4/3 -> Sum1/3
  [u_S3abc] -> Product1/1
  Demux4/2 -> Sum1/2
  Product1/1 -> Demux4/1
  u_Sab/1 -> ab0 - ABC/1(BPu)
  [u_S3abc] -> u_S3abc/1
  [i_S3abc] -> i_S3abc/1
  ab0 - ABC/1(u) -> [u_S3abc]
  ab0 - ABC1/1(u) -> [i_S3abc]
  IIR Filter/1 -> Product2/1, Demux1/1
  RMS/1 -> Scope11/1
  Demux1/2 -> u_S3abc1/2
  Demux1/3 -> u_S3abc1/3
  Demux1/1 -> RMS/1, u_S3abc1/1
  From1/1 -> IIR Filter/1
  Demux2/1 -> RMS1/1, i_S3abc1/1
  RMS1/1 -> Scope1/1
  Demux2/2 -> i_S3abc1/2
  IIR Filter1/1 -> Product2/2, Demux2/1
  From2/1 -> IIR Filter1/1
  Demux2/3 -> i_S3abc1/3
  Demux3/2 -> Sum2/2
  Demux3/3 -> Sum2/3
  Sum2/1 -> Scope/1
  Product2/1 -> Demux3/1
  Demux3/1 -> Sum2/1

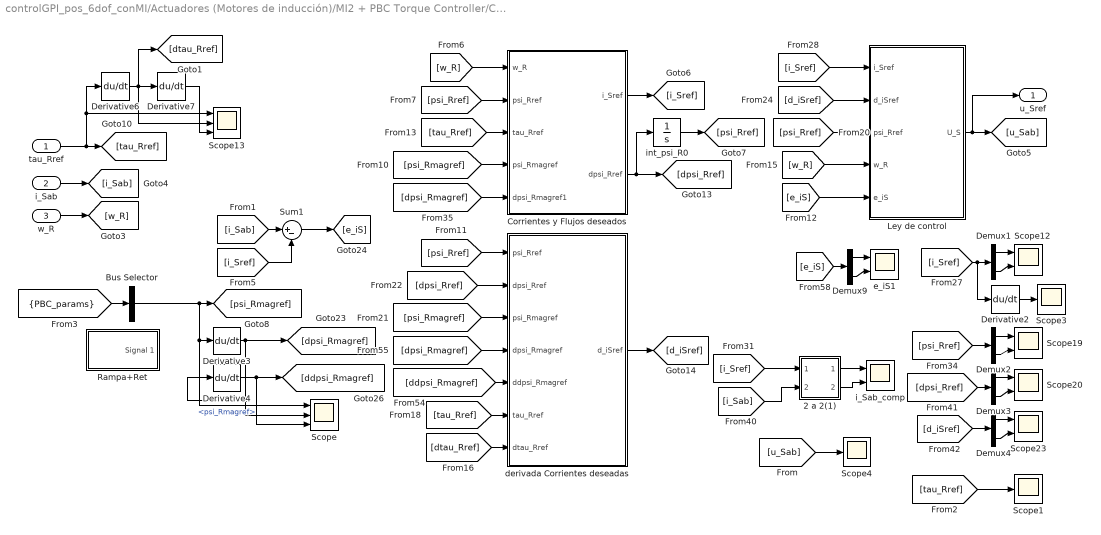
== system controlGPI_pos_6dof_conMI/Actuadores (Motores de inducción)/MI2 + PBC Torque Controller/Controlador PBC ==
  tau_Rref : Inport
  i_Sab : Inport  Port=2
  w_R : Inport  Port=3
  2 a 2(1) : Subsystem
  Bus Selector : BusSelector  OutputSignals=psi_Rmagref
  Corrientes y Flujos deseados : Subsystem
  Demux{1..4,9} (5 alike) : Demux  Outputs=2
  Derivative{2..4,6..7} (5 alike) : Derivative
  Ley de control : Subsystem
  Rampa+Ret : Subsystem  Tag=STV Subsys  LoadFcn=sigbuilder_block('load');  StartFcn=sigbuilder_block('start');  StopFcn=sigbuilder_block('stop');  ClipboardFcn=sigbuilder_block('clipboard');  mask(Sigbuilder block){tuvar=[0:10]}
      mask help: Sigbuilder GUI
      mask init:
      | if ~strcmp(get_param(bdroot(gcbh),'SimulationStatus'),'stopped') tuvar = sigbuilder_block('maskInit'); end
      settings: CopyFcn=sigbuilder_block('copy');  DeleteFcn=sigbuilder_block('delete');  ModelCloseFcn=sigbuilder_block('modelClose');  PreSaveFcn=sigbuilder_block('preSave');  PauseFcn=sigbuilder_block('pause')  ContinueFcn=sigbuilder_block('continue')  NameChangeFcn=sigbuilder_block('namechange');  OpenFcn=sigbuilder_block('open',[280.5 86.5 550.5 399.5 ]);  CloseFcn=sigbuilder_block('close');
      mask Display: plot(0, 0, 100, 100,[2, 2, 32, 32, 2], [68, 8, 8, 68, 68],[32, 2], [38, 38], [32, 19, 2],[53, 60, 44], [32, 17, 17, 2],[16, 16, 31, 31]);txt = getActiveGroup(gcbh);text(2, 100, txt,'verticalAlignment', 'top');
  Scope : Scope  NumInputPorts=3
  Scope1 : Scope
  Scope{12,19..20,23} (4 alike) : Scope  NumInputPorts=2
  Scope13 : Scope  NumInputPorts=3
  Scope3 : Scope
  Scope4 : Scope
  Sum1 : Sum  Inputs=|+-
  derivada Corrientes deseadas : Subsystem
  e_iS1 : Scope  NumInputPorts=2
  i_Sab_comp : Scope  NumInputPorts=2
  int_psi_R0 : Integrator  InitialCondition=[1.1675;0]
  u_Sref : Outport
  wires:
  Derivative3/1 -> Scope/2, Derivative4/1, [dpsi_Rmagref]
  Derivative4/1 -> [ddpsi_Rmagref], Scope/3
  Bus Selector/1 -> Scope/1, Derivative3/1, [psi_Rmagref]  "<psi_Rmagref>"
  i_Sab/1 -> [i_Sab]
  Demux1/1 -> Scope12/1
  [d_iSref] -> Demux4/1
  Demux3/2 -> Scope20/2
  Demux2/1 -> Scope19/1
  Demux1/2 -> Scope12/2
  [dpsi_Rref] -> Demux3/1
  Demux3/1 -> Scope20/1
  Demux4/1 -> Scope23/1
  [psi_Rref] -> Demux2/1
  Demux4/2 -> Scope23/2
  Demux2/2 -> Scope19/2
  [tau_Rref] -> Corrientes y Flujos deseados/3(tau_Rref)
  [w_R] -> Corrientes y Flujos deseados/1(w_R)
  int_psi_R0/1 -> [psi_Rref]
  Corrientes y Flujos deseados/2(dpsi_Rref) -> int_psi_R0/1, [dpsi_Rref]
  [psi_Rref] -> Corrientes y Flujos deseados/2(psi_Rref)
  [psi_Rmagref] -> Corrientes y Flujos deseados/4(psi_Rmagref)
  [dpsi_Rmagref] -> Corrientes y Flujos deseados/5(dpsi_Rmagref1)
  [psi_Rref] -> derivada Corrientes deseadas/1(psi_Rref)
  [dpsi_Rref] -> derivada Corrientes deseadas/2(dpsi_Rref)
  [psi_Rmagref] -> derivada Corrientes deseadas/3(psi_Rmagref)
  [dpsi_Rmagref] -> derivada Corrientes deseadas/4(dpsi_Rmagref)
  [ddpsi_Rmagref] -> derivada Corrientes deseadas/5(ddpsi_Rmagref)
  [tau_Rref] -> derivada Corrientes deseadas/6(tau_Rref)
  [dtau_Rref] -> derivada Corrientes deseadas/7(dtau_Rref)
  derivada Corrientes deseadas/1(d_iSref) -> [d_iSref]
  [e_iS] -> Demux9/1
  Demux9/1 -> e_iS1/1
  Demux9/2 -> e_iS1/2
  [i_Sab] -> Sum1/1
  [i_Sref] -> Sum1/2
  Sum1/1 -> [e_iS]
  [u_Sab] -> Scope4/1
  [i_Sref] -> Ley de control/1(i_Sref)
  [d_iSref] -> Ley de control/2(d_iSref)
  [psi_Rref] -> Ley de control/3(psi_Rref)
  [w_R] -> Ley de control/4(w_R)
  Ley de control/1(U_S) -> u_Sref/1, [u_Sab]
  [e_iS] -> Ley de control/5(e_iS)
  Derivative7/1 -> Scope13/3
  tau_Rref/1 -> Derivative6/1, Scope13/1, [tau_Rref]
  Derivative6/1 -> [dtau_Rref], Derivative7/1, Scope13/2
  2 a 2(1)/2(Out2) -> i_Sab_comp/2
  2 a 2(1)/1(Out1) -> i_Sab_comp/1
  [i_Sab] -> 2 a 2(1)/2(In2)
  [i_Sref] -> 2 a 2(1)/1(In1)
  [i_Sref] -> Derivative2/1, Demux1/1
  Derivative2/1 -> Scope3/1
  w_R/1 -> [w_R]
  [tau_Rref] -> Scope1/1
  [PBC_params] -> Bus Selector/1
  Corrientes y Flujos deseados/1(i_Sref) -> [i_Sref]

== system controlGPI_pos_6dof_conMI/Actuadores (Motores de inducción)/MI2 + PBC Torque Controller/Modelo MI (Subsistema eléctrico) ==
  u_Sab : Inport
  tau_L : Inport  Port=2
  w_R : Inport  Port=3
  Demux : Demux  Outputs=2
  Demux7 : Demux  Outputs=2
  Demux8 : Demux  Outputs=2
  Integrator : Integrator
  Integrator1 : Integrator
  Modelo Motor de inducción (Subsistema eléctrico) : MATLAB Function  TreatAsAtomicUnit=on
  Scope11 : Scope
  Scope3 : Scope  NumInputPorts=2
  Scope31 : Scope
  ab/dq : MATLAB Function  TreatAsAtomicUnit=on
  d_iSab : Scope  NumInputPorts=2
  dpsi_Rab1 : Scope  NumInputPorts=2
  i_Sab : Outport
  psi_Rab : Outport  Port=2
  tau_R : Outport  Port=3
  wires:
  Modelo Motor de inducción (Subsistema eléctrico)/1(di_Sab) -> Integrator/1, [d_iSab]
  Modelo Motor de inducción (Subsistema eléctrico)/2(dpsi_Rab) -> Integrator1/1, [dpsi_Rab]
  [w_R] -> Modelo Motor de inducción (Subsistema eléctrico)/5(w_R)
  [psi_Rab] -> Modelo Motor de inducción (Subsistema eléctrico)/4(psi_Rab)
  [i_Sab] -> Modelo Motor de inducción (Subsistema eléctrico)/3(i_Sab)
  Integrator1/1 -> [psi_Rab]
  u_Sab/1 -> [u_Sab]
  Modelo Motor de inducción (Subsistema eléctrico)/3(tau_R) -> [tau_R]
  [tau_R] -> Scope3/1
  ab/dq/1(psi_Rmag) -> Scope11/1
  [psi_Rab] -> Demux/1
  Demux7/1 -> dpsi_Rab1/1
  Demux7/2 -> dpsi_Rab1/2
  [d_iSab] -> Demux8/1
  ab/dq/2(rho) -> Scope31/1
  Demux/1 -> ab/dq/1(psi_ra)
  Demux8/2 -> d_iSab/2
  Demux8/1 -> d_iSab/1
  [dpsi_Rab] -> Demux7/1
  Demux/2 -> ab/dq/2(psi_rb)
  Integrator/1 -> [i_Sab]
  [MI_motor_params] -> Modelo Motor de inducción (Subsistema eléctrico)/1(MI_motor_params)
  [u_Sab] -> Modelo Motor de inducción (Subsistema eléctrico)/2(u_Sab)
  tau_L/1 -> [tau_L]
  [tau_L] -> Modelo Motor de inducción (Subsistema eléctrico)/6(tau_L)
  w_R/1 -> [w_R]
  [tau_R] -> tau_R/1
  [psi_Rab] -> psi_Rab/1
  [i_Sab] -> i_Sab/1
  [tau_L] -> Scope3/2

== system controlGPI_pos_6dof_conMI/Actuadores (Motores de inducción)/MI3 + PBC Torque Controller/Calculo de Potencia eléctrica ==
  u_Sab : Inport
  i_Sab : Inport  Port=2
  Demux1 : Demux  Commented=on  Outputs=3
  Demux2 : Demux  Commented=on  Outputs=3
  Demux3 : Demux  Commented=on  Outputs=3
  Demux4 : Demux  Outputs=3
  From1 : From  Commented=on  GotoTag=u_S3abc
  From2 : From  Commented=on  GotoTag=i_S3abc
  IIR Filter : mcbcontrolslib/IIR Filter  Commented=on  VariantControl=Low Pass Filter  VariantSelect=Low-pass  Filter_constant=0.04  advancedSettings=on  Ts=50e-6  cutOff_freq=132.6291
      settings: LibrarySourceBlock=mcbhdllib/Signal Management/IIR Filter
  IIR Filter1 : mcbcontrolslib/IIR Filter  Commented=on  VariantControl=Low Pass Filter  VariantSelect=Low-pass  Filter_constant=0.04  advancedSettings=on  Ts=50e-6  cutOff_freq=132.6291
      settings: LibrarySourceBlock=mcbhdllib/Signal Management/IIR Filter
  Product1 : Product
  Product2 : Product  Commented=on
  RMS : spsRMSLib/RMS  Commented=on  TrueRMS=on  Freq=60  RMSInit=120  Ts=0
  RMS1 : spsRMSLib/RMS  Commented=on  TrueRMS=on  Freq=60  RMSInit=120  Ts=0
  Scope : Scope  Commented=on
  Scope1 : Scope  Commented=on
  Scope11 : Scope  Commented=on
  Sum1 : Sum  Inputs=|+++
  Sum2 : Sum  Commented=on  Inputs=|+++
  ab0 - ABC : MATLAB Function  TreatAsAtomicUnit=on
  ab0 - ABC1 : MATLAB Function  TreatAsAtomicUnit=on
  i_S3abc1 : Scope  Commented=on  NumInputPorts=3
  u_S3abc1 : Scope  Commented=on  NumInputPorts=3
  P_elect : Outport
  u_S3abc : Outport  Port=2
  i_S3abc : Outport  Port=3
  wires:
  Sum1/1 -> P_elect/1
  Demux4/1 -> Sum1/1
  [i_S3abc] -> Product1/2
  i_Sab/1 -> ab0 - ABC1/1(BPu)
  Demux4/3 -> Sum1/3
  [u_S3abc] -> Product1/1
  Demux4/2 -> Sum1/2
  Product1/1 -> Demux4/1
  u_Sab/1 -> ab0 - ABC/1(BPu)
  [u_S3abc] -> u_S3abc/1
  [i_S3abc] -> i_S3abc/1
  ab0 - ABC/1(u) -> [u_S3abc]
  ab0 - ABC1/1(u) -> [i_S3abc]
  IIR Filter/1 -> Product2/1, Demux1/1
  RMS/1 -> Scope11/1
  Demux1/2 -> u_S3abc1/2
  Demux1/3 -> u_S3abc1/3
  Demux1/1 -> RMS/1, u_S3abc1/1
  From1/1 -> IIR Filter/1
  Demux2/1 -> RMS1/1, i_S3abc1/1
  RMS1/1 -> Scope1/1
  Demux2/2 -> i_S3abc1/2
  IIR Filter1/1 -> Product2/2, Demux2/1
  From2/1 -> IIR Filter1/1
  Demux2/3 -> i_S3abc1/3
  Demux3/2 -> Sum2/2
  Demux3/3 -> Sum2/3
  Sum2/1 -> Scope/1
  Product2/1 -> Demux3/1
  Demux3/1 -> Sum2/1
